simulink model "SingleJoint_Algorithm2"  (R2018b)
settings: Solver=FixedStepDiscrete  StartTime=0.0  StopTime=Inf  FixedStep=0.001  RelTol=1e-3  EnableMultiTasking=on
undefined symbols (not defined in the file): DiscIntNeverNeededParam, J3, J7, Motor_Current, Motor_Position, Motor_Velocity, Send_GUIdata
libraries: c280xlib x14, simulink x7, dspsrcs4 x1, idelinklib_common x1
(part 1 of 2)
settings Model: ExtModeTrigDuration=8  Creator=jeason  LastModifiedBy=Jeason
settings SolverCC: AutoInsertRateTranBlk=on
settings OptimizationCC: DefaultUnderspecifiedDataType=single  EnhancedBackFolding=on  PassReuseOutputArgsAs=Individual arguments  MaxStackSize=512  OptimizeBlockOrder=speed  DifferentSizesBufferReuse=on  OptimizationCustomize=off
settings DebuggingCC: MultiTaskDSMMsg=none  ParameterTunabilityLossMsg=error
settings HardwareCC: ProdBitPerChar=16  ProdBitPerInt=16  ProdBitPerPointer=32  ProdBitPerSizeT=32  ProdBitPerPtrDiffT=32  ProdLargestAtomicInteger=Integer  ProdLargestAtomicFloat=None  ProdWordSize=16  ProdLongLongMode=on  ProdHWDeviceType=Texas Instruments->C2000
settings SFSimCC: MATLABDynamicMemAlloc=off
settings RTWCC: SystemTargetFile=ert.tlc  HardwareBoard=TI Delfino F2833x  TemplateMakefile=ert_default_tmf  GenerateReport=on  Toolchain=Texas Instruments Code Composer Studio (C2000)  IncludeHyperlinkInReport=on  LaunchReport=on  GenerateTraceInfo=on  GenerateTraceReport=on  GenerateTraceReportSl=on  GenerateTraceReportSf=on  GenerateTraceReportEml=on
settings CodeAppCC: ForceParamTrailComments=on  IgnoreCustomStorageClasses=off  OperatorAnnotations=on  SimulinkDataObjDesc=on  SFDataObjDesc=on  InsertBlockDesc=on
settings ERTTargetCC: CodeReplacementLibrary=TI C28x

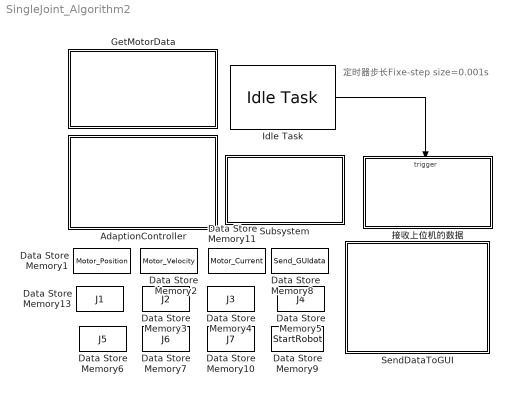
== system SingleJoint_Algorithm2 ==
  note: 定时器步长Fixe-step size=0.001s
  AdaptionController : Subsystem  Tag=Calculated_Data  Priority=1  TreatAsAtomicUnit=on  RTWFcnName=DynamicsController
      settings: RTWSystemCode=Nonreusable function  RTWFcnNameOpts=User specified  RTWFileNameOpts=Use function name
      mask Display:
      | color('red')
      | disp('六轴单关节\n自适应算法2动力学计算')
  Data Store Memory1 : DataStoreMemory  DataStoreName=Motor_Position  ReadBeforeWriteMsg=warning  WriteAfterWriteMsg=warning  WriteAfterReadMsg=warning  InitialValue=[0 0 0 0 0 0]  ShowAdditionalParam=off  OutDataTypeStr=int32
      settings: RTWStateStorageClass=ExportedGlobal
  Data Store Memory10 : DataStoreMemory  DataStoreName=J7  ReadBeforeWriteMsg=warning  WriteAfterWriteMsg=warning  WriteAfterReadMsg=warning  InitialValue=[0 0 0 0 0 0]  ShowAdditionalParam=off  OutDataTypeStr=double
      settings: RTWStateStorageClass=ExportedGlobal
  Data Store Memory11 : DataStoreMemory  DataStoreName=Motor_Current  ReadBeforeWriteMsg=warning  WriteAfterWriteMsg=warning  WriteAfterReadMsg=warning  InitialValue=[0 0 0 0 0 0]  ShowAdditionalParam=off  OutDataTypeStr=int32
      settings: RTWStateStorageClass=ExportedGlobal
  Data Store Memory13 : DataStoreMemory  DataStoreName=J1  ReadBeforeWriteMsg=warning  WriteAfterWriteMsg=warning  WriteAfterReadMsg=warning  InitialValue=[0 0 0 0 0 0]  ShowAdditionalParam=off  OutDataTypeStr=double
      settings: RTWStateStorageClass=ExportedGlobal
  Data Store Memory2 : DataStoreMemory  DataStoreName=Motor_Velocity  ReadBeforeWriteMsg=warning  WriteAfterWriteMsg=warning  WriteAfterReadMsg=warning  InitialValue=[0 0 0 0 0 0]  ShowAdditionalParam=off  OutDataTypeStr=int32
      settings: RTWStateStorageClass=ExportedGlobal
  Data Store Memory3 : DataStoreMemory  DataStoreName=J2  ReadBeforeWriteMsg=warning  WriteAfterWriteMsg=warning  WriteAfterReadMsg=warning  InitialValue=[0 0 0 0 0 0]  ShowAdditionalParam=off  OutDataTypeStr=double
      settings: RTWStateStorageClass=ExportedGlobal
  Data Store Memory4 : DataStoreMemory  DataStoreName=J3  ReadBeforeWriteMsg=warning  WriteAfterWriteMsg=warning  WriteAfterReadMsg=warning  InitialValue=[0 0 0 0 0 0]  ShowAdditionalParam=off  OutDataTypeStr=double
      settings: RTWStateStorageClass=ExportedGlobal
  Data Store Memory5 : DataStoreMemory  DataStoreName=J4  ReadBeforeWriteMsg=warning  WriteAfterWriteMsg=warning  WriteAfterReadMsg=warning  InitialValue=[0 0 0 0 0 0]  ShowAdditionalParam=off  OutDataTypeStr=double
      settings: RTWStateStorageClass=ExportedGlobal
  Data Store Memory6 : DataStoreMemory  DataStoreName=J5  ReadBeforeWriteMsg=warning  WriteAfterWriteMsg=warning  WriteAfterReadMsg=warning  InitialValue=[0 0 0 0 0 0]  ShowAdditionalParam=off  OutDataTypeStr=double
      settings: RTWStateStorageClass=ExportedGlobal
  Data Store Memory7 : DataStoreMemory  DataStoreName=J6  ReadBeforeWriteMsg=warning  WriteAfterWriteMsg=warning  WriteAfterReadMsg=warning  InitialValue=[0 0 0 0 0 0]  ShowAdditionalParam=off  OutDataTypeStr=double
      settings: RTWStateStorageClass=ExportedGlobal
  Data Store Memory8 : DataStoreMemory  DataStoreName=Send_GUIdata  ReadBeforeWriteMsg=warning  WriteAfterWriteMsg=warning  WriteAfterReadMsg=warning  InitialValue=zeros(1,18)  ShowAdditionalParam=off  OutDataTypeStr=double
      settings: RTWStateStorageClass=ExportedGlobal
  Data Store Memory9 : DataStoreMemory  DataStoreName=StartRobot  ReadBeforeWriteMsg=warning  WriteAfterWriteMsg=warning  WriteAfterReadMsg=warning  ShowAdditionalParam=off  OutDataTypeStr=uint16
      settings: RTWStateStorageClass=ExportedGlobal
  GetMotorData : Subsystem  Tag=Get_Data  Priority=0  TreatAsAtomicUnit=on
      settings: RTWSystemCode=Nonreusable function
  Idle Task : idelinklib_common/Idle Task  tasknumbers=[0]  taskpriorities=100016  taskpreempts=[1]  showinput=off  simPriority=0
  SendDataToGUI : Subsystem  Priority=2  TreatAsAtomicUnit=on
      settings: RTWSystemCode=Nonreusable function
  Subsystem : Subsystem
      mask Display: disp('System\nInitialization');
  接收上位机的数据 : Subsystem  TreatAsAtomicUnit=on
  wires:
  Idle Task/1 -> 接收上位机的数据/Trigger

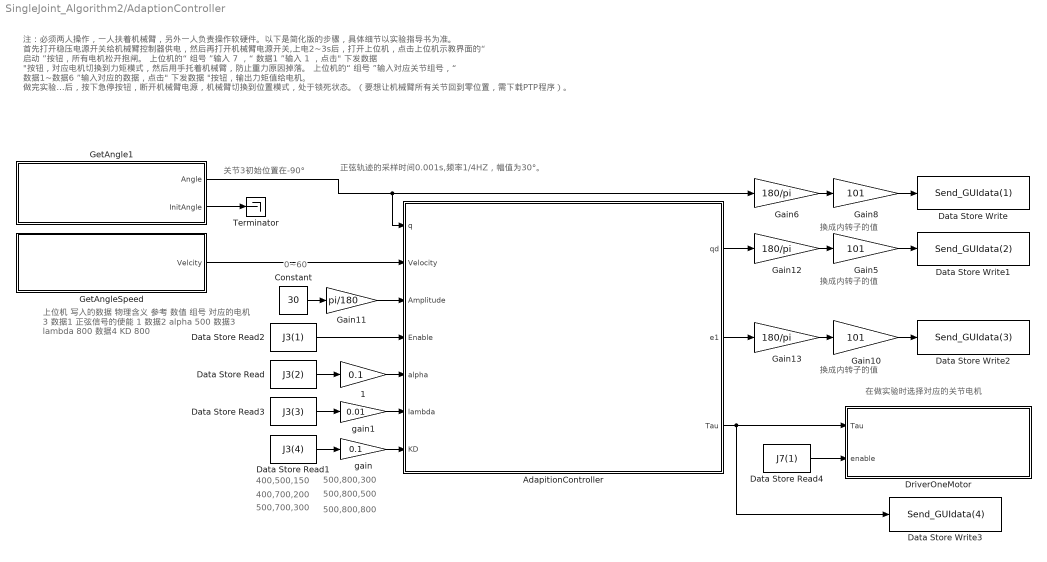
== system SingleJoint_Algorithm2/AdaptionController ==
  note: 400,500,150
  note: 换成内转子的值
  note: 换成内转子的值
  note: 换成内转子的值
  note: 在做实验时选择对应的关节电机
  note: 上位机
      | 写入的数据
      | 物理含义
      | 参考
      | 数值
      |
      | 组号
      | 对应的电机
      | 3
      |
      | 数据1
      | 正弦信号的使能
      | 1
      |
      | 数据2
      | alpha
      | 500
      |
      | 数据3
      | lambda
      | 800
      |
      | 数据4
      | KD
      | 800
  note: 关节3初始位置在-90°
  note: 400,700,200
  note: 500,700,300
  note: 500,800,300
  note: 500,800,800
  note: 注：必须两人操作，一人扶着机械臂，另外一人负责操作软硬件。以下是简化版的步骤，具体细节以实验指导书为准。
      | 首先打开稳压电源开关给机械臂控制器供电，然后再打开机械臂电源开关,上电2~3s后，打开上位机，点击上位机示教界面的“ 启动 ”按钮，所有电机松开抱闸。
      | 上位机的“ 组号 ”输入 7 ，“ 数据1 ”输入 1 ，点击" 下发数据 "按钮，对应电机切换到力矩模式，然后用手托着机械臂，防止重力原因掉落。
      | 上位机的“ 组号 ”输入对应关节组号，“ 数据1~数据6 ”输入对应的数据，点击" 下发数据 "按钮，输出力矩值给电机。
      | 做完实验后，按下急停按钮，断开机械臂电源，机械臂切换到位置模式，处于锁死状态。（要想让机械臂所有关节回到零位置，需下载PTP程序）。
  note: 500,800,500
  note: 正弦轨迹的采样时间0.001s,频率1/4HZ，幅值为30°。
  note: 0~60
  1 : Gain  Gain=0.1  OutDataTypeStr=double
  AdapitionController : Subsystem  Priority=2  TreatAsAtomicUnit=on  RTWFcnName=AdaptiveAlgorithm  mask(单关节自适应算法2控制器){Freq=1/4, SimpleTime=0.001}
      mask prompts: Freq "正弦信号的频率(HZ)"; SimpleTime "正弦信号的采样时间(s)"
      mask help:
      | 采样频率不能过快，否则机械臂摆动频率也会变快，至少为1/4.
      | 采样时间只能是定时器步长的整数倍，否则会报错，正弦信号的幅值最大为pi/3。
      settings: RTWSystemCode=Nonreusable function  RTWFcnNameOpts=User specified  RTWFileNameOpts=Use subsystem name  FunctionInterfaceSpec=Allow arguments
      mask Display:
      | port_label('input', 1, '外转子实际角度(rad)');
      | port_label('input', 2, '外转子实际角速度(rad/s)');
      | port_label('input', 3, '外转子正弦信号的幅值(rad)');
      | port_label('input', 4, '使能信号');
      | port_label('input', 5, 'alpha');
      | port_label('input', 6, 'lambda');
      | port_label('input', 7, 'KD');
      | 
      | port_label('output', 1, '外转子理想正弦信号(rad)');
      | port_label('output', 2, '外转子跟踪误差(rad)');
      | port_label('output', 3, '力矩Tau(N·m)');
  Constant : Constant  Value=30
  Data Store Read : DataStoreRead  DataStoreName=J3  DataStoreElements=J3(2)
  Data Store Read1 : DataStoreRead  DataStoreName=J3  DataStoreElements=J3(4)
  Data Store Read2 : DataStoreRead  DataStoreName=J3  DataStoreElements=J3(1)
  Data Store Read3 : DataStoreRead  DataStoreName=J3  DataStoreElements=J3(3)
  Data Store Read4 : DataStoreRead  DataStoreName=J7  DataStoreElements=J7(1)
  Data Store Write : DataStoreWrite  DataStoreName=Send_GUIdata  DataStoreElements=Send_GUIdata(1)
  Data Store Write1 : DataStoreWrite  DataStoreName=Send_GUIdata  DataStoreElements=Send_GUIdata(2)
  Data Store Write2 : DataStoreWrite  DataStoreName=Send_GUIdata  DataStoreElements=Send_GUIdata(3)
  Data Store Write3 : DataStoreWrite  DataStoreName=Send_GUIdata  DataStoreElements=Send_GUIdata(4)
  DriverOneMotor : Subsystem  TreatAsAtomicUnit=on  mask(驱动单个关节){SelectJoint=3}
      mask prompts: SelectJoint "选择关节电机"
      mask help:
      | 关节1~3为CANB,关节4~6为CANA,驱动的电机的邮箱号统一为7。
      | 输入量的范围限定在-900~900。
      settings: RTWSystemCode=Nonreusable function
      mask TypeOptions SelectJoint: 1 | 2 | 3 | 4 | 5 | 6
      mask Callback SelectJoint:
      | vssBlk1_1 = [gcb, '/BottomDriver/Joint1'];
      | vssBlk1_2 = [gcb, '/BottomDriver/Joint2'];
      | vssBlk1_3 = [gcb, '/BottomDriver/Joint3'];
      | vssBlk1_4 = [gcb, '/BottomDriver/Joint4'];
      | vssBlk1_5 = [gcb, '/BottomDriver/Joint5'];
      | vssBlk1_6 = [gcb, '/BottomDriver/Joint6'];
      | choice1 = get_param(gcb,'SelectJoint');
      | if strcmp(choice1,'1')
      |     set_param(vssBlk1_1, 'Commented','off');
      |     set_param(vssBlk1_2,'Commented','on');
      |     set_param(vssBlk1_3,'Commented','on');
      |     set_param(vssBlk1_4,'Commented','on');
      |     set_param(vssBlk1_5,'Commented','on');
      |     set_param(vssBlk1_6,'Commented','on');
      | elseif strcmp(choice1,'2')
      |     set_param(vssBlk1_2, 'Commented','off');
      |     set_param(vssBlk1_1,'Commented','on');
      |     set_param(vssBlk1_3,'Commented','on');
      |     set_param(vssBlk1_4,'Commented','on');
      |     set_param(vssBlk1_5,'Commented','on');
      |     set_param(vssBlk1_6,'Commented','on');
      | elseif strcmp(choice1,'3')
      |     set_param(vssBlk1_3, 'Commented','off');
      |     set_param(vssBlk1_1,'Commented','on');
      |     set_param(vssBlk1_2,'Commented','on');
      |     set_param(vssBlk1_4,'Commented','on');
      |     set_param(vssBlk1_5,'Commented','on');
      |     set_param(vssBlk1_6,'Commented','on');
      | elseif strcmp(choice1,'4')
      |     set_param(vssBlk1_4, 'Commented','off');
      |     set_param(vssBlk1_1,'Commented','on');
      |     set_param(vssBlk1_2,'Commented','on');
      |     set_param(vssBlk1_3,'Commented','on');
      |     set_param(vssBlk1_5,'Commented','on');
      |     set_param(vssBlk1_6,'Commented','on');
      | elseif strcmp(choice1,'5')
      |     set_param(vssBlk1_5, 'Commented','off');
      |     set_param(vssBlk1_1,'Commented','on');
      |     set_param(vssBlk1_2,'Commented','on');
      |     set_param(vssBlk1_3,'Commented','on');
      |     set_param(vssBlk1_4,'Commented','on');
      |     set_param(vssBlk1_6,'Commented','on');
      | elseif strcmp(choice1,'6')
      |     set_param(vssBlk1_6, 'Commented','off');
      |     set_param(vssBlk1_1,'Commented','on');
      |     set_param(vssBlk1_2,'Commented','on');
      |     set_param(vssBlk1_3,'Commented','on');
      |     set_param(vssBlk1_4,'Commented','on');
      |     set_param(vssBlk1_5,'Commented','on');
      | end
      | clear choice1 vssBlk1_1 vssBlk1_2 vssBlk1_3 vssBlk1_4 vssBlk1_5 vssBlk1_6;
      mask Display:
      | port_label('input', 1, 'Tau');
      | port_label('input', 2, 'Enable');
      | choice1 = get_param(gcb,'SelectJoint');
      | color('black');
      | switch choice1
      |     case '1'
      |         disp('单关节算法\n驱动关节1电机');
      |     case '2'
      |         disp('单关节算法\n驱动关节2电机');
      |     case '3'
      |         disp('单关节算法\n驱动关节3电机');
      |     case '4'
      |         disp('单关节算法\n驱动关节4电机');
      |     case '5'
      |         disp('单关节算法\n驱动关节5电机');
      |     case '6'
      |         disp('单关节算法\n驱动关节6电机');
      | end
      | clear choice1;
  Gain10 : Gain  Gain=101
  Gain11 : Gain  Gain=pi/180
  Gain12 : Gain  Gain=180/pi  OutDataTypeStr=double
  Gain13 : Gain  Gain=180/pi  OutDataTypeStr=double
  Gain5 : Gain  Gain=101
  Gain6 : Gain  Gain=180/pi  OutDataTypeStr=double
  Gain8 : Gain  Gain=101
  GetAngle1 : Subsystem  TreatAsAtomicUnit=on  mask(获取电机外转子角度(rad)){JJoint=3, InitAngle=-90}
      mask prompts: JJoint "选择关节电机"; InitAngle "给定初始角度(deg)"
      mask help:
      | 给定初始角度：假设在数学建模时，设定连杆在水平位置为0°，而机械臂每个关节在出厂时都设定在竖直位置为0°，那么这里就需要给定一个偏置值90°/-90°，默认设为0。
      | 注：关节3因为结构原因实际获取到的角度的正负和标签贴的方向相反。
      | Angle(rad)=电机外转子的实际角度值-给定的初始角度值
      | InitAngle(rad)=给定的初始角度值
      mask TypeOptions JJoint: 1 | 2 | 3 | 4 | 5 | 6
      mask Display:
      | choice1 = get_param(gcb,'JJoint');
      | color('black');
      | switch choice1
      |     case '1'
      |         disp('获取关节1电机\n外转子角度(rad)');
      |     case '2'
      |         disp('获取关节2电机\n外转子角度(rad)');
      |     case '3'
      |         disp('获取关节3电机\n外转子角度(rad)');
      |     case '4'
      |         disp('获取关节4电机\n外转子角度(rad)');
      |     case '5'
      |         disp('获取关节5电机\n外转子角度(rad)');
      |     case '6'
      |         disp('获取关节6电机\n外转子角度(rad)');
      | end
      | color('black');
      | port_label('output', 1, 'Angle');
      | port_label('output', 2, 'InitAngle');
      | clear choice1;
  GetAngleSpeed : Subsystem  Priority=2  TreatAsAtomicUnit=on  mask{JJoint=3}
      mask prompts: JJoint "选择关节电机"
      mask help: 读取电机角速度(rad/s)
      mask TypeOptions JJoint: 1 | 2 | 3 | 4 | 5 | 6
      mask Display:
      | choice1 = get_param(gcb,'JJoint');
      | color('black');
      | switch choice1
      |     case '1'
      |         disp('获取关节1电机\n外转子角速度(rad/s)');
      |     case '2'
      |         disp('获取关节2电机\n外转子角速度(rad/s)');
      |     case '3'
      |         disp('获取关节3电机\n外转子角速度(rad/s)');
      |     case '4'
      |         disp('获取关节4电机\n外转子角速度(rad/s)');
      |     case '5'
      |         disp('获取关节5电机\n外转子角速度(rad/s)');
      |     case '6'
      |         disp('获取关节6电机\n外转子角速度(rad/s)');
      | end
      | color('black');
      | port_label('output', 1, 'Velocity');
      | clear choice1;
  Terminator : Terminator
  gain : Gain  Gain=0.1  OutDataTypeStr=double
  gain1 : Gain  Gain=0.01  OutDataTypeStr=double
  wires:
  GetAngle1/1(Angle) -> AdapitionController/1(q), Gain6/1
  Gain10/1 -> Data Store Write2/1
  Gain5/1 -> Data Store Write1/1
  Data Store Read/1 -> 1/1
  Data Store Read3/1 -> gain1/1
  Data Store Read1/1 -> gain/1
  Gain6/1 -> Gain8/1
  Gain8/1 -> Data Store Write/1
  Constant/1 -> Gain11/1
  Gain12/1 -> Gain5/1
  Gain13/1 -> Gain10/1
  GetAngleSpeed/1(Velcity) -> AdapitionController/2(Velocity)
  1/1 -> AdapitionController/5(alpha)
  Data Store Read2/1 -> AdapitionController/4(Enable)
  Gain11/1 -> AdapitionController/3(Amplitude)
  gain1/1 -> AdapitionController/6(lambda)
  gain/1 -> AdapitionController/7(KD)
  AdapitionController/1(qd) -> Gain12/1
  AdapitionController/2(e1) -> Gain13/1
  Data Store Read4/1 -> DriverOneMotor/2(enable)
  AdapitionController/3(Tau) -> DriverOneMotor/1(Tau), Data Store Write3/1
  GetAngle1/2(InitAngle) -> Terminator/1

== system SingleJoint_Algorithm2/GetMotorData ==
  note: 获取关节电流、 角速度、 角度信息
  CANA_284_24 : Subsystem  Priority=4  TreatAsAtomicUnit=on
      settings: RTWSystemCode=Nonreusable function
      mask Display:
      | color('WHITE')
      | disp('JOINT4\n数据读取')
  CANA_285_25 : Subsystem  Priority=5  TreatAsAtomicUnit=on
      settings: RTWSystemCode=Nonreusable function
      mask Display:
      | color('WHITE')
      | disp('JOINT5\n数据读取')
  CANA_286_26 : Subsystem  Priority=6  TreatAsAtomicUnit=on
      settings: RTWSystemCode=Nonreusable function
      mask Display:
      | color('WHITE')
      | disp('JOINT6\n数据读取')
  CANB_281_21 : Subsystem  Priority=1  TreatAsAtomicUnit=on
      settings: RTWSystemCode=Nonreusable function
      mask Display:
      | color('WHITE')
      | disp('JOINT1\n数据读取')
  CANB_282_22 : Subsystem  Priority=2  TreatAsAtomicUnit=on
      settings: RTWSystemCode=Nonreusable function
      mask Display:
      | color('white')
      | disp('JOINT2\n数据读取')
  CANB_283_23 : Subsystem  Priority=3  TreatAsAtomicUnit=on
      settings: RTWSystemCode=Nonreusable function
      mask Display:
      | color('white')
      | disp('JOINT3\n数据读取')

== system SingleJoint_Algorithm2/SendDataToGUI ==
  note: Upper limit=9
  note: 发送数据给上位机
  note: 定时器步长Fixe-step size=0.001s,
      | 每10ms发送一次数据给上位机
  " " : Subsystem
  Constant : Constant  Value=true  OutDataTypeStr=boolean
  Constant1 : Constant  Value=false  OutDataTypeStr=boolean
  Switch : Switch  Criteria=u2 > Threshold
  广播周期 : simulink/Sources/Counter Limited  uplimit=9  tsamp=-1
  wires:
  Switch/1 -> " "/Enable
  广播周期/1 -> Switch/2
  Constant1/1 -> Switch/1
  Constant/1 -> Switch/3

== system SingleJoint_Algorithm2/Subsystem ==
  Model Header : Subsystem  mask(Model Header){ShowInLibBrowser=0}
      mask prompts: ShowInLibBrowser "Simulink:masks:CustCodeMaskParam1_MP"
      settings: CopyFcn=cccopyfcn(gcb)  OpenFcn=ccopenfcn('Model Header')
      mask Help: eval('feval(''rtwprivate'',''rtwhelpview'',''rtw_model_header_block'')');
      mask Display: disp('Model\nHeader');
  Model Source : Subsystem  mask(Model Source){ShowInLibBrowser=0}
      mask prompts: ShowInLibBrowser "Simulink:masks:CustCodeMaskParam1_MP"
      settings: CopyFcn=cccopyfcn(gcb)  OpenFcn=ccopenfcn('Model Source')
      mask Help: eval('feval(''rtwprivate'',''rtwhelpview'',''rtw_model_source_block'')');
      mask Display: disp('Model\nSource');
  System Initialize : Subsystem  mask(System Initialize){ShowInLibBrowser=0}
      mask prompts: ShowInLibBrowser "Simulink:masks:CustCodeMaskParam1_MP"
      settings: CopyFcn=cccopyfcn(gcb)  OpenFcn=ccopenfcn('System Initialize Function')
      mask Help: eval('feval(''rtwprivate'',''rtwhelpview'',''rtw_sys_initialize_block'')');
      mask Display: disp('System\nInitialize');

== system SingleJoint_Algorithm2/接收上位机的数据 ==
  note: 接收上位机数据
  function : TriggerPort  TriggerType=function-call  VariantControl=Variant
  0x0080 : simulink/Logic and Bit Operations/Compare To Constant  relop===  const=hex2dec('0080')  OutDataTypeStr=boolean
  0x88 : simulink/Logic and Bit Operations/Compare To Constant  relop===  const=hex2dec('0088')  OutDataTypeStr=boolean
  Compare To Constant1 : simulink/Logic and Bit Operations/Compare To Constant  relop===  const=hex2dec('0001')  OutDataTypeStr=boolean
  Compare To Constant2 : simulink/Logic and Bit Operations/Compare To Constant  relop===  const=hex2dec('0001')  OutDataTypeStr=boolean
  Data Store Read : DataStoreRead  DataStoreName=PTX
  Data Store Write2 : DataStoreWrite  DataStoreName=StartRobot
  Data Type Conversion : DataTypeConversion  OutDataTypeStr=int16
  Data Type Conversion3 : DataTypeConversion  OutDataTypeStr=double
  Data Type Conversion4 : DataTypeConversion  OutDataTypeStr=uint16
  Demux1 : Demux  Outputs=9
  Logical Operator : Logic  Inputs=4  AllPortsSameDT=off  OutDataTypeStr=boolean
  Mux1 : Mux  Inputs=6
  Subsystem : Subsystem
  Terminator3 : Terminator
  消息使能 : DataStoreMemory  DataStoreName=PTX  ReadBeforeWriteMsg=warning  WriteAfterWriteMsg=warning  WriteAfterReadMsg=warning  InitialValue=true  ShowAdditionalParam=off  OutDataTypeStr=boolean
  获取用户命令 : Subsystem  Priority=1  TreatAsAtomicUnit=on
      settings: RTWSystemCode=Nonreusable function
  wires:
  Compare To Constant2/1 -> Logical Operator/4
  Compare To Constant1/1 -> Logical Operator/3
  Data Store Read/1 -> Logical Operator/2
  Logical Operator/1 -> Data Type Conversion4/1
  0x0080/1 -> Logical Operator/1
  Demux1/4 -> Mux1/2, Compare To Constant2/1
  Demux1/3 -> Mux1/1, Compare To Constant1/1
  Demux1/1 -> 0x0080/1, 0x88/1
  获取用户命令/1(消息) -> Demux1/1
  Demux1/5 -> Mux1/3
  Demux1/6 -> Mux1/4
  Demux1/9 -> Terminator3/1
  Demux1/7 -> Mux1/5
  Demux1/8 -> Mux1/6
  Mux1/1 -> Data Type Conversion/1
  Data Type Conversion/1 -> Data Type Conversion3/1
  Data Type Conversion4/1 -> Data Store Write2/1
  Demux1/2 -> Subsystem/1(组号)
  Data Type Conversion3/1 -> Subsystem/2(数据)
  0x88/1 -> Subsystem/Enable

== system SingleJoint_Algorithm2/AdaptionController/AdapitionController ==
  q : Inport
  Velocity : Inport  Port=2
  Amplitude : Inport  Port=3
  Enable : Inport  Port=4
  alpha : Inport  Port=5
  lambda : Inport  Port=6
  KD : Inport  Port=7
  Controller : Subsystem  TreatAsAtomicUnit=on
      settings: RTWSystemCode=Nonreusable function
  Error : Subsystem  TreatAsAtomicUnit=on
      settings: RTWSystemCode=Nonreusable function
  Terminator1 : Terminator
  Terminator2 : Terminator
  限幅 : Saturate  UpperLimit=pi/3  LowerLimit=0
  qd : Outport
  e1 : Outport  Port=2
  Tau : Outport  Port=3
  wires:
  Velocity/1 -> Controller/2(velocity), Error/2(velocity)
  Error/2(e1) -> e1/1
  alpha/1 -> Error/5(alpha)
  Error/1(qd) -> qd/1
  Amplitude/1 -> 限幅/1
  Error/6(d_theta_r) -> Terminator1/1
  Error/5(V) -> Terminator2/1
  Enable/1 -> Error/3(enable)
  q/1 -> Controller/1(position), Error/1(q)
  Error/3(dd_theta_r) -> Controller/3(dd_theta_r)
  Error/4(s) -> Controller/4(s)
  lambda/1 -> Controller/5(lambda)
  KD/1 -> Controller/6(KD)
  Controller/1(tau) -> Tau/1
  限幅/1 -> Error/4(gain)

== system SingleJoint_Algorithm2/AdaptionController/DriverOneMotor ==
  note: CAN mbx=7
  Tau : Inport
  enable : Inport  Port=2
  BottomDriver : Subsystem
  Constant1 : Constant  Value=SelectJoint
  Data Store Memory2 : DataStoreMemory  DataStoreName=One_TXD  ReadBeforeWriteMsg=warning  WriteAfterWriteMsg=warning  WriteAfterReadMsg=warning  InitialValue=[0]  ShowAdditionalParam=off  OutDataTypeStr=uint8
      settings: RTWStateStorageClass=ExportedGlobal
  Data Store Read4 : DataStoreRead  DataStoreName=One_TXD
  限幅 : Saturate  UpperLimit=500  LowerLimit=-500
  驱动器指令 : Subsystem  TreatAsAtomicUnit=on
      settings: RTWSystemCode=Nonreusable function
  wires:
  Data Store Read4/1 -> BottomDriver/Enable
  Constant1/1 -> BottomDriver/1(SelectJoint)
  驱动器指令/1(MSG) -> BottomDriver/2(MSG)
  限幅/1 -> 驱动器指令/1(Current)
  Tau/1 -> 限幅/1
  enable/1 -> 驱动器指令/2(enable)

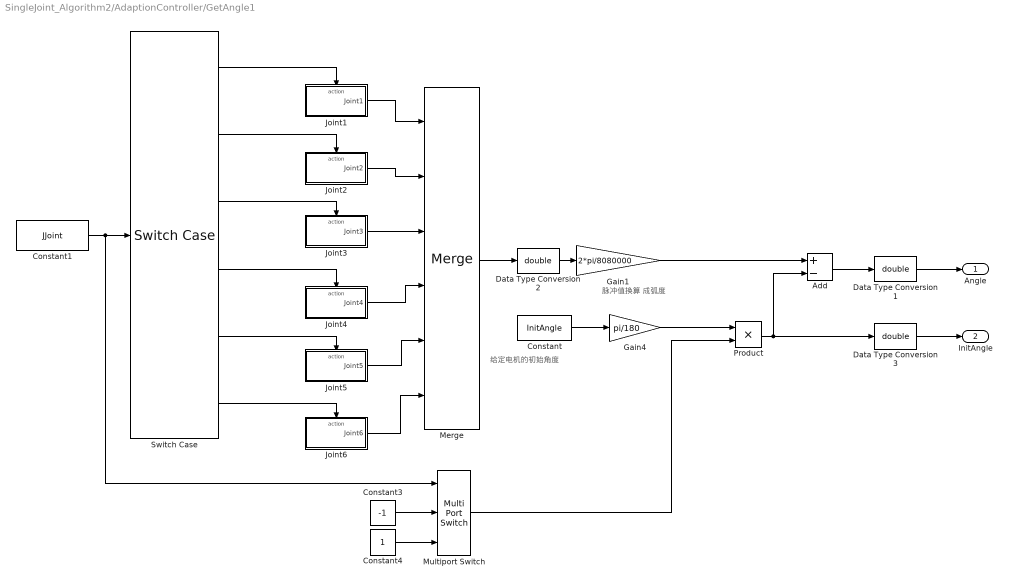
== system SingleJoint_Algorithm2/AdaptionController/GetAngle1 ==
  note: 脉冲值换算
      | 成弧度
  note: 给定电机的初始角度
  Add : Sum  Inputs=+-
  Constant : Constant  Value=InitAngle
  Constant1 : Constant  Value=JJoint  OutDataTypeStr=uint8
  Constant3 : Constant  Value=-1
  Constant4 : Constant
  Data Type Conversion1 : DataTypeConversion  OutDataTypeStr=double
  Data Type Conversion2 : DataTypeConversion  OutDataTypeStr=double
  Data Type Conversion3 : DataTypeConversion  OutDataTypeStr=double
  Gain1 : Gain  Gain=2*pi/8080000
  Gain4 : Gain  Gain=pi/180
  Joint1 : Subsystem  TreatAsAtomicUnit=on
  Joint2 : Subsystem  TreatAsAtomicUnit=on
  Joint3 : Subsystem  TreatAsAtomicUnit=on
  Joint4 : Subsystem  TreatAsAtomicUnit=on
  Joint5 : Subsystem  TreatAsAtomicUnit=on
  Joint6 : Subsystem  TreatAsAtomicUnit=on
  Merge : Merge  Inputs=6  InitialOutput=0
  Multiport Switch : MultiPortSwitch  DataPortOrder=Specify indices  Inputs=2  DataPortIndices={3,[1,2,4,5,6]}
  Product : Product
  Switch Case : SwitchCase  CaseConditions={1 2 3 4 5 6}  ShowDefaultCase=off
  Angle : Outport
  InitAngle : Outport  Port=2
  wires:
  Data Type Conversion2/1 -> Gain1/1
  Data Type Conversion1/1 -> Angle/1
  Joint6/1(Joint6) -> Merge/6
  Joint5/1(Joint5) -> Merge/5
  Joint4/1(Joint4) -> Merge/4
  Joint3/1(Joint3) -> Merge/3
  Joint2/1(Joint2) -> Merge/2
  Joint1/1(Joint1) -> Merge/1
  Switch Case/6 -> Joint6/Action
  Switch Case/5 -> Joint5/Action
  Switch Case/4 -> Joint4/Action
  Switch Case/3 -> Joint3/Action
  Switch Case/2 -> Joint2/Action
  Switch Case/1 -> Joint1/Action
  Constant/1 -> Gain4/1
  Add/1 -> Data Type Conversion1/1
  Gain1/1 -> Add/1
  Gain4/1 -> Product/1
  Merge/1 -> Data Type Conversion2/1
  Multiport Switch/1 -> Product/2
  Constant4/1 -> Multiport Switch/3
  Constant3/1 -> Multiport Switch/2
  Constant1/1 -> Multiport Switch/1, Switch Case/1
  Product/1 -> Data Type Conversion3/1, Add/2
  Data Type Conversion3/1 -> InitAngle/1

== system SingleJoint_Algorithm2/AdaptionController/GetAngleSpeed ==
  note: 换算成角速度2π/1min
  Constant1 : Constant  Value=JJoint
  Data Type Conversion3 : DataTypeConversion  OutDataTypeStr=double
  Gain3 : Gain  Gain=2*pi/60
  Gain9 : Gain  Gain=1/101
  Joint1 : Subsystem  TreatAsAtomicUnit=on
  Joint2 : Subsystem  TreatAsAtomicUnit=on
  Joint3 : Subsystem  TreatAsAtomicUnit=on
  Joint4 : Subsystem  TreatAsAtomicUnit=on
  Joint5 : Subsystem  TreatAsAtomicUnit=on
  Joint6 : Subsystem  TreatAsAtomicUnit=on
  Merge1 : Merge  Inputs=6  InitialOutput=0
  Switch Case : SwitchCase  CaseConditions={1 2 3 4 5 6}  ShowDefaultCase=off
  Velcity : Outport
  wires:
  Constant1/1 -> Switch Case/1
  Switch Case/1 -> Joint1/Action
  Switch Case/2 -> Joint2/Action
  Switch Case/3 -> Joint3/Action
  Switch Case/4 -> Joint4/Action
  Switch Case/5 -> Joint5/Action
  Switch Case/6 -> Joint6/Action
  Data Type Conversion3/1 -> Gain3/1
  Joint6/1(Joint6_Velocity) -> Merge1/6
  Joint5/1(Joint5_Velocity) -> Merge1/5
  Joint4/1(Joint4_Velocity) -> Merge1/4
  Joint3/1(Joint3_Velocity) -> Merge1/3
  Joint2/1(Joint2_Velocity) -> Merge1/2
  Joint1/1(Joint1_Velocity) -> Merge1/1
  Gain3/1 -> Gain9/1
  Gain9/1 -> Velcity/1
  Merge1/1 -> Data Type Conversion3/1

== system SingleJoint_Algorithm2/GetMotorData/CANA_284_24 ==
  note: 控制器接收ID:0x280+“ID”
  Subsystem1 : Subsystem
  eCAN Receive1 : c280xlib/eCAN Receive  chipFamily=C280x  useModule=eCAN_A  mailboxNo=24  messageID=hex2dec('284')  messageType=Standard (11-bit identifier)  sampleTime=-1  dataType=uint8  initValue=0  outputMessageLength=off  outputMessageTimeStamp=off  postInterrupt=off  interruptLine=0
      settings: SourceProductName=Embedded Coder Support Package for Texas Instruments C2000 Processors  SourceProductBaseCode=TIC2000
  wires:
  eCAN Receive1/2 -> Subsystem1/1(In1)
  eCAN Receive1/1 -> Subsystem1/Trigger

== system SingleJoint_Algorithm2/GetMotorData/CANA_285_25 ==
  note: 控制器接收ID:0x280+“ID”
  Subsystem : Subsystem
  eCAN Receive : c280xlib/eCAN Receive  chipFamily=C280x  useModule=eCAN_A  mailboxNo=25  messageID=hex2dec('285')  messageType=Standard (11-bit identifier)  sampleTime=-1  dataType=uint8  initValue=0  outputMessageLength=off  outputMessageTimeStamp=off  postInterrupt=off  interruptLine=0
      settings: SourceProductName=Embedded Coder Support Package for Texas Instruments C2000 Processors  SourceProductBaseCode=TIC2000
  wires:
  eCAN Receive/2 -> Subsystem/1(In1)
  eCAN Receive/1 -> Subsystem/Trigger

== system SingleJoint_Algorithm2/GetMotorData/CANA_286_26 ==
  note: 控制器接收ID:0x280+“ID”
  Subsystem : Subsystem
  eCAN Receive : c280xlib/eCAN Receive  chipFamily=C280x  useModule=eCAN_A  mailboxNo=26  messageID=hex2dec('286')  messageType=Standard (11-bit identifier)  sampleTime=-1  dataType=uint8  initValue=0  outputMessageLength=off  outputMessageTimeStamp=off  postInterrupt=off  interruptLine=0
      settings: SourceProductName=Embedded Coder Support Package for Texas Instruments C2000 Processors  SourceProductBaseCode=TIC2000
  wires:
  eCAN Receive/2 -> Subsystem/1(In1)
  eCAN Receive/1 -> Subsystem/Trigger

== system SingleJoint_Algorithm2/GetMotorData/CANB_281_21 ==
  note: 控制器接收ID:0x280+“ID”
  Subsystem : Subsystem
  eCAN Receive : c280xlib/eCAN Receive  chipFamily=C280x  useModule=eCAN_B  mailboxNo=21  messageID=hex2dec('281')  messageType=Standard (11-bit identifier)  sampleTime=-1  dataType=uint8  initValue=0  outputMessageLength=off  outputMessageTimeStamp=off  postInterrupt=off  interruptLine=0
      settings: SourceProductName=Embedded Coder Support Package for Texas Instruments C2000 Processors  SourceProductBaseCode=TIC2000
  wires:
  eCAN Receive/2 -> Subsystem/1(In1)
  eCAN Receive/1 -> Subsystem/Trigger

== system SingleJoint_Algorithm2/GetMotorData/CANB_282_22 ==
  note: 控制器接收ID:0x280+“ID”
  Subsystem : Subsystem
  eCAN Receive : c280xlib/eCAN Receive  chipFamily=C280x  useModule=eCAN_B  mailboxNo=22  messageID=hex2dec('282')  messageType=Standard (11-bit identifier)  sampleTime=-1  dataType=uint8  initValue=0  outputMessageLength=off  outputMessageTimeStamp=off  postInterrupt=off  interruptLine=0
      settings: SourceProductName=Embedded Coder Support Package for Texas Instruments C2000 Processors  SourceProductBaseCode=TIC2000
  wires:
  eCAN Receive/2 -> Subsystem/1(In1)
  eCAN Receive/1 -> Subsystem/Trigger

== system SingleJoint_Algorithm2/GetMotorData/CANB_283_23 ==
  note: 控制器接收ID:0x280+“ID”
  Subsystem : Subsystem
  eCAN Receive : c280xlib/eCAN Receive  chipFamily=C280x  useModule=eCAN_B  mailboxNo=23  messageID=hex2dec('283')  messageType=Standard (11-bit identifier)  sampleTime=-1  dataType=uint8  initValue=0  outputMessageLength=off  outputMessageTimeStamp=off  postInterrupt=off  interruptLine=0
      settings: SourceProductName=Embedded Coder Support Package for Texas Instruments C2000 Processors  SourceProductBaseCode=TIC2000
  wires:
  eCAN Receive/2 -> Subsystem/1(In1)
  eCAN Receive/1 -> Subsystem/Trigger

== system SingleJoint_Algorithm2/SendDataToGUI/  ==
  Enable : EnablePort
  Constant1 : Constant  Value=hex2dec('5a')  OutDataTypeStr=uint16
  Data Store Read4 : DataStoreRead  DataStoreName=Send_GUIdata
  Data Type Conversion12 : DataTypeConversion  OutDataTypeStr=uint16
  Demux : Demux  Outputs=18
  Mux : Mux  Inputs=20
  SCI Transmit : c280xlib/SCI Transmit  sciModule=A  dataHead=''  dataTail=''  postInterrupt=off  numFifo=1
      settings: SourceProductName=Embedded Coder Support Package for Texas Instruments C2000 Processors
  校验码填充 : Sum  Inputs=+++++++++++++++++++  AccumDataTypeStr=uint16
  wires:
  Demux/1 -> Mux/2, 校验码填充/2
  Mux/1 -> SCI Transmit/1
  Demux/3 -> 校验码填充/4, Mux/4
  Demux/14 -> 校验码填充/15, Mux/15
  Demux/9 -> 校验码填充/10, Mux/10
  Demux/5 -> Mux/6, 校验码填充/6
  Demux/2 -> 校验码填充/3, Mux/3
  Data Store Read4/1 -> Data Type Conversion12/1
  Demux/13 -> 校验码填充/14, Mux/14
  Demux/6 -> Mux/7, 校验码填充/7
  Demux/8 -> 校验码填充/9, Mux/9
  Demux/10 -> 校验码填充/11, Mux/11
  Demux/4 -> 校验码填充/5, Mux/5
  Demux/7 -> 校验码填充/8, Mux/8
  Demux/15 -> 校验码填充/16, Mux/16
  Demux/11 -> 校验码填充/12, Mux/12
  Demux/18 -> 校验码填充/19, Mux/19
  Demux/16 -> 校验码填充/17, Mux/17
  Constant1/1 -> 校验码填充/1, Mux/1
  Demux/17 -> 校验码填充/18, Mux/18
  校验码填充/1 -> Mux/20
  Demux/12 -> 校验码填充/13, Mux/13
  Data Type Conversion12/1 -> Demux/1

== system SingleJoint_Algorithm2/Subsystem/Model Header ==

== system SingleJoint_Algorithm2/Subsystem/Model Source ==

== system SingleJoint_Algorithm2/Subsystem/System Initialize ==

== system SingleJoint_Algorithm2/接收上位机的数据/Subsystem ==
  组号 : Inport
  数据 : Inport  Port=2
  Enable : EnablePort
  Joint1 : Subsystem  TreatAsAtomicUnit=on
  Joint2 : Subsystem  TreatAsAtomicUnit=on
  Joint3 : Subsystem  TreatAsAtomicUnit=on
  Joint4 : Subsystem  TreatAsAtomicUnit=on
  Joint5 : Subsystem  TreatAsAtomicUnit=on
  Joint6 : Subsystem  TreatAsAtomicUnit=on
  Joint7 : Subsystem  TreatAsAtomicUnit=on
  Switch Case : SwitchCase  CaseConditions={1 2 3 4 5 6 7}  ShowDefaultCase=off
  wires:
  数据/1 -> Joint7/1(Joint7), Joint5/1(Joint5), Joint4/1(Joint4), Joint3/1(Joint3), Joint2/1(Joint2), Joint1/1(Joint1), Joint6/1(Joint6)
  Switch Case/5 -> Joint5/Action
  Switch Case/6 -> Joint6/Action
  Switch Case/2 -> Joint2/Action
  Switch Case/1 -> Joint1/Action
  Switch Case/3 -> Joint3/Action
  Switch Case/4 -> Joint4/Action
  组号/1 -> Switch Case/1
  Switch Case/7 -> Joint7/Action

== system SingleJoint_Algorithm2/接收上位机的数据/获取用户命令 ==
  " " : c280xlib/SCI Receive  sciModule=A  dataHead=''  dataTail=''  dataType=uint16  dataDim=9  initValue=0  errOption=Output the last received value  errValue=0  sampleTime=-1  outputStatus=on  postInterrupt=off  numFifo=1
      settings: SourceProductName=Embedded Coder Support Package for Texas Instruments C2000 Processors  SourceProductBaseCode=TIC2000
  Constant : Constant  Value=false  OutDataTypeStr=boolean
  Constant1 : Constant  Value=true  OutDataTypeStr=boolean
  Data Store Write1 : DataStoreWrite  DataStoreName=PTX
  Logical Operator : Logic  AllPortsSameDT=off  OutDataTypeStr=boolean
  Switch : Switch  Criteria=u2 > Threshold
  消息校验 : Subsystem
  消息 : Outport
  wires:
  消息校验/2(使能) -> Logical Operator/1
  Switch/1 -> Logical Operator/2
  Constant1/1 -> Switch/3
  " "/2 -> Switch/2
  消息校验/1(消息) -> 消息/1
  " "/1 -> 消息校验/1(数据)
  Logical Operator/1 -> Data Store Write1/1
  Constant/1 -> Switch/1

== system SingleJoint_Algorithm2/AdaptionController/AdapitionController/Controller ==
  note: $\dot \eta_2=F\eta_2+HY(\theta,\dot\theta,\ddot\theta_r)+FHY_J(s)$
  note: $\dot \eta_1=F\eta_1+H\tau$
  note: $\tau=f\hat\omega+\Gamma_0\eta_1-K_Ds$
  note: 延时一个采样周期
  position : Inport
  velocity : Inport  Port=2
  dd_theta_r : Inport  Port=3
  s : Inport  Port=4
  lambda : Inport  Port=5
  KD : Inport  Port=6
  Discrete-Time Integrator1 : DiscreteIntegrator  SampleTime=-1  LimitOutput=on  UpperSaturationLimit=[1000 1000 1000;1000 1000 1000;1000 1000 1000;]  LowerSaturationLimit=[-1000 -1000 -1000;-1000 -1000 -1000;-1000 -1000 -1000;]  ICPrevOutput=DiscIntNeverNeededParam  ICPrevScaledInput=DiscIntNeverNeededParam
  Discrete-Time Integrator3 : DiscreteIntegrator  SampleTime=-1  LimitOutput=on  UpperSaturationLimit=[1000;1000;1000;]  LowerSaturationLimit=[-1000;-1000;-1000;]  ICPrevOutput=DiscIntNeverNeededParam  ICPrevScaledInput=DiscIntNeverNeededParam
  SolveTau : Subsystem  TreatAsAtomicUnit=on
      settings: RTWSystemCode=Nonreusable function  FunctionInterfaceSpec=Allow arguments
  Unit Delay : UnitDelay  SampleTime=-1
  Unit Delay1 : UnitDelay  SampleTime=-1
  Unit Delay2 : UnitDelay  SampleTime=-1
  adaptive : Subsystem  TreatAsAtomicUnit=on
      settings: RTWSystemCode=Nonreusable function  FunctionInterfaceSpec=Allow arguments
  im1 : Subsystem  TreatAsAtomicUnit=on
      settings: RTWSystemCode=Nonreusable function  FunctionInterfaceSpec=Allow arguments
  im2 : Subsystem  TreatAsAtomicUnit=on
      settings: RTWSystemCode=Nonreusable function  FunctionInterfaceSpec=Allow arguments
  tau : Outport
  wires:
  im2/1(d_eta2) -> Discrete-Time Integrator1/1
  Unit Delay1/1 -> adaptive/1(eta1), im1/2(eta1)
  s/1 -> im2/4(s), SolveTau/5(s), adaptive/6(s)
  dd_theta_r/1 -> im2/3(dd_theta_r), adaptive/5(dd_theta_r)
  position/1 -> adaptive/3(theta), im2/1(position)
  Discrete-Time Integrator1/1 -> Unit Delay2/1
  Discrete-Time Integrator3/1 -> Unit Delay1/1
  Unit Delay/1 -> im1/1(tau)
  im1/1(d_eta1) -> Discrete-Time Integrator3/1
  Unit Delay2/1 -> adaptive/2(eta2), im2/5(eta2)
  velocity/1 -> adaptive/4(d_theta), im2/2(d_theta)
  SolveTau/1(Tau) -> Unit Delay/1, tau/1
  adaptive/1(Gamma0 eta1) -> SolveTau/1(Gamma0 eta1)
  adaptive/2(f) -> SolveTau/2(f)
  lambda/1 -> SolveTau/3(lambda)
  KD/1 -> SolveTau/4(KD)

== system SingleJoint_Algorithm2/AdaptionController/AdapitionController/Error ==
  note: 期望速度
  note: 期望位置
  note: $s(t)=\alpha e_1(t)+e_2(t)$
  note: $\dot\theta_r(t)=\dot\theta_d(t)-\alpha e_1(t)$
  note: $\ddot\theta_r(t)=\ddot\theta_d(t)-\alpha e_2(t)$
  note: $e_2(t)=\dot\theta(t)-\dot\theta_d(t)$
  q : Inport
  velocity : Inport  Port=2
  enable : Inport  Port=3
  gain : Inport  Port=4
  alpha : Inport  Port=5
  Discrete Derivative : simulink/Discrete/Discrete Derivative  gainval=1.0  ICPrevScaledInput=0.0  OutMin=[]  OutMax=[]  OutDataType=fixdt(1, 16)  OutScaling=2^-10  DoSatur=off
  Discrete Derivative1 : simulink/Discrete/Discrete Derivative  gainval=1.0  ICPrevScaledInput=0.0  OutMin=[]  OutMax=[]  OutDataType=fixdt(1, 16)  OutScaling=2^-10  DoSatur=off
  Product1 : Product
  Product5 : Product
  Subsystem : Subsystem
  Sum1 : Sum  Inputs=|-+
  Sum2 : Sum  Inputs=|-+
  Sum3 : Sum  Inputs=|-+
  Sum4 : Sum  Inputs=++|
  qd : Outport
  e1 : Outport  Port=2
  dd_theta_r : Outport  Port=3
  s : Outport  Port=4
  V : Outport  Port=5
  d_theta_r : Outport  Port=6
  wires:
  velocity/1 -> Sum1/2
  Product1/1 -> Sum4/1, Sum2/1
  Sum1/1 -> Product5/2, Sum4/2
  Product5/1 -> Sum3/1
  Sum2/1 -> d_theta_r/1
  Sum3/1 -> dd_theta_r/1
  Sum4/1 -> s/1
  enable/1 -> Subsystem/Enable
  Discrete Derivative/1 -> Sum2/2, V/1, Sum1/1, Discrete Derivative1/1
  Discrete Derivative1/1 -> Sum3/2
  alpha/1 -> Product1/2, Product5/1
  Subsystem/2(qd) -> qd/1, Discrete Derivative/1
  Subsystem/1(e1) -> e1/1, Product1/1
  q/1 -> Subsystem/1(q1)
  gain/1 -> Subsystem/2(gian)

== system SingleJoint_Algorithm2/AdaptionController/DriverOneMotor/BottomDriver ==
  SelectJoint : Inport
  MSG : Inport  Port=2
  Enable : EnablePort
  Joint1 : Subsystem  Commented=on  TreatAsAtomicUnit=on
  Joint2 : Subsystem  Commented=on  TreatAsAtomicUnit=on
  Joint3 : Subsystem  TreatAsAtomicUnit=on
  Joint4 : Subsystem  Commented=on  TreatAsAtomicUnit=on
  Joint5 : Subsystem  Commented=on  TreatAsAtomicUnit=on
  Joint6 : Subsystem  Commented=on  TreatAsAtomicUnit=on
  Switch Case : SwitchCase  CaseConditions={1 2 3 4 5 6}  ShowDefaultCase=off
  wires:
  SelectJoint/1 -> Switch Case/1
  Switch Case/6 -> Joint6/Action
  Switch Case/4 -> Joint4/Action
  Switch Case/2 -> Joint2/Action
  Switch Case/1 -> Joint1/Action
  Switch Case/3 -> Joint3/Action
  Switch Case/5 -> Joint5/Action
  MSG/1 -> Joint1/1(In6), Joint3/1(In1), Joint6/1(In1), Joint5/1(In1), Joint4/1(In1), Joint2/1(In1)

== system SingleJoint_Algorithm2/AdaptionController/DriverOneMotor/驱动器指令 ==
  Current : Inport
  enable : Inport  Port=2
  Data Store Read : DataStoreRead  DataStoreName=StartRobot
  Data Type Conversion1 : DataTypeConversion  OutDataTypeStr=uint8
  Data Type Conversion4 : DataTypeConversion  OutDataTypeStr=uint16
  Data Type Conversion7 : DataTypeConversion  OutDataTypeStr=uint16
  DriveOder : Stateflow chart  TreatAsAtomicUnit=on
  MSG : Outport  OutDataTypeStr=uint8
  wires:
  Data Type Conversion7/1 -> DriveOder/1(Current)
  Current/1 -> Data Type Conversion7/1
  DriveOder/1(MSG) -> Data Type Conversion1/1
  Data Type Conversion1/1 -> MSG/1
  Data Store Read/1 -> DriveOder/2(StartRobot)
  Data Type Conversion4/1 -> DriveOder/3(write)
  enable/1 -> Data Type Conversion4/1

== system SingleJoint_Algorithm2/AdaptionController/GetAngle1/Joint1 ==
  note: 内转子位置的脉冲值
  Action Port : ActionPort
  Data Store Read5 : DataStoreRead  DataStoreName=Motor_Position  DataStoreElements=Motor_Position(1)
  Joint1 : Outport
  wires:
  Data Store Read5/1 -> Joint1/1

== system SingleJoint_Algorithm2/AdaptionController/GetAngle1/Joint2 ==
  Action Port : ActionPort
  Data Store Read5 : DataStoreRead  DataStoreName=Motor_Position  DataStoreElements=Motor_Position(2)
  Joint2 : Outport
  wires:
  Data Store Read5/1 -> Joint2/1

== system SingleJoint_Algorithm2/AdaptionController/GetAngle1/Joint3 ==
  Action Port : ActionPort
  Data Store Read5 : DataStoreRead  DataStoreName=Motor_Position  DataStoreElements=Motor_Position(3)
  Joint3 : Outport
  wires:
  Data Store Read5/1 -> Joint3/1

== system SingleJoint_Algorithm2/AdaptionController/GetAngle1/Joint4 ==
  Action Port : ActionPort
  Data Store Read5 : DataStoreRead  DataStoreName=Motor_Position  DataStoreElements=Motor_Position(4)
  Joint4 : Outport
  wires:
  Data Store Read5/1 -> Joint4/1

== system SingleJoint_Algorithm2/AdaptionController/GetAngle1/Joint5 ==
  Action Port : ActionPort
  Data Store Read5 : DataStoreRead  DataStoreName=Motor_Position  DataStoreElements=Motor_Position(5)
  Joint5 : Outport
  wires:
  Data Store Read5/1 -> Joint5/1

== system SingleJoint_Algorithm2/AdaptionController/GetAngle1/Joint6 ==
  Action Port : ActionPort
  Data Store Read5 : DataStoreRead  DataStoreName=Motor_Position  DataStoreElements=Motor_Position(6)
  Joint6 : Outport
  wires:
  Data Store Read5/1 -> Joint6/1

== system SingleJoint_Algorithm2/AdaptionController/GetAngleSpeed/Joint1 ==
  note: 内转子速度
      | 的脉冲值
  Action Port : ActionPort  ActionType=case
  Data Store Read1 : DataStoreRead  DataStoreName=Motor_Velocity  DataStoreElements=Motor_Velocity(1)
  Joint1_Velocity : Outport
  wires:
  Data Store Read1/1 -> Joint1_Velocity/1

== system SingleJoint_Algorithm2/AdaptionController/GetAngleSpeed/Joint2 ==
  note: 内转子速度
      | 的脉冲值
  Action Port : ActionPort  ActionType=case
  Data Store Read1 : DataStoreRead  DataStoreName=Motor_Velocity  DataStoreElements=Motor_Velocity(2)
  Joint2_Velocity : Outport
  wires:
  Data Store Read1/1 -> Joint2_Velocity/1

== system SingleJoint_Algorithm2/AdaptionController/GetAngleSpeed/Joint3 ==
  note: 内转子速度
      | 的脉冲值
  Action Port : ActionPort  ActionType=case
  Data Store Read1 : DataStoreRead  DataStoreName=Motor_Velocity  DataStoreElements=Motor_Velocity(3)
  Joint3_Velocity : Outport
  wires:
  Data Store Read1/1 -> Joint3_Velocity/1

== system SingleJoint_Algorithm2/AdaptionController/GetAngleSpeed/Joint4 ==
  note: 内转子速度
      | 的脉冲值
  Action Port : ActionPort  ActionType=case
  Data Store Read1 : DataStoreRead  DataStoreName=Motor_Velocity  DataStoreElements=Motor_Velocity(4)
  Joint4_Velocity : Outport
  wires:
  Data Store Read1/1 -> Joint4_Velocity/1

== system SingleJoint_Algorithm2/AdaptionController/GetAngleSpeed/Joint5 ==
  note: 内转子速度
      | 的脉冲值
  Action Port : ActionPort  ActionType=case
  Data Store Read1 : DataStoreRead  DataStoreName=Motor_Velocity  DataStoreElements=Motor_Velocity(5)
  Joint5_Velocity : Outport
  wires:
  Data Store Read1/1 -> Joint5_Velocity/1

== system SingleJoint_Algorithm2/AdaptionController/GetAngleSpeed/Joint6 ==
  note: 内转子速度
      | 的脉冲值
  Action Port : ActionPort  ActionType=case
  Data Store Read1 : DataStoreRead  DataStoreName=Motor_Velocity  DataStoreElements=Motor_Velocity(6)
  Joint6_Velocity : Outport
  wires:
  Data Store Read1/1 -> Joint6_Velocity/1

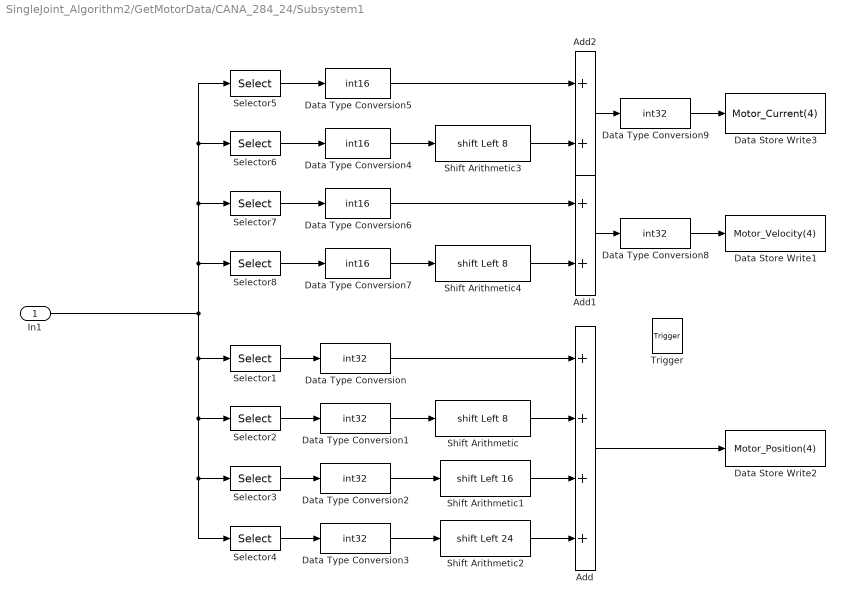
== system SingleJoint_Algorithm2/GetMotorData/CANA_284_24/Subsystem1 ==
  In1 : Inport
  Trigger : TriggerPort  TriggerType=function-call  VariantControl=Variant  PortDimensions=1
  Add : Sum  Inputs=4
  Add1 : Sum  Inputs=2
  Add2 : Sum  Inputs=2
  Data Store Write1 : DataStoreWrite  DataStoreName=Motor_Velocity  DataStoreElements=Motor_Velocity(4)
  Data Store Write2 : DataStoreWrite  DataStoreName=Motor_Position  DataStoreElements=Motor_Position(4)
  Data Store Write3 : DataStoreWrite  DataStoreName=Motor_Current  DataStoreElements=Motor_Current(4)
  Data Type Conversion{,1..3,8..9} (6 alike) : DataTypeConversion  OutDataTypeStr=int32
  Data Type Conversion{4..7} (4 alike) : DataTypeConversion  OutDataTypeStr=int16
  Selector1 : Selector  IndexMode=Zero-based  InputPortWidth=8  IndexOptions=Index vector (dialog)  Indices=4  OutputSizes=1
  Selector2 : Selector  IndexMode=Zero-based  InputPortWidth=8  IndexOptions=Index vector (dialog)  Indices=5  OutputSizes=1
  Selector3 : Selector  IndexMode=Zero-based  InputPortWidth=8  IndexOptions=Index vector (dialog)  Indices=6  OutputSizes=1
  Selector4 : Selector  IndexMode=Zero-based  InputPortWidth=8  IndexOptions=Index vector (dialog)  Indices=7  OutputSizes=1
  Selector5 : Selector  IndexMode=Zero-based  InputPortWidth=8  IndexOptions=Index vector (dialog)  Indices=0  OutputSizes=1
  Selector6 : Selector  IndexMode=Zero-based  InputPortWidth=8  IndexOptions=Index vector (dialog)  Indices=1  OutputSizes=1
  Selector7 : Selector  IndexMode=Zero-based  InputPortWidth=8  IndexOptions=Index vector (dialog)  Indices=2  OutputSizes=1
  Selector8 : Selector  IndexMode=Zero-based  InputPortWidth=8  IndexOptions=Index vector (dialog)  Indices=3  OutputSizes=1
  Shift Arithmetic : ArithShift  BitShiftNumber=8  BitShiftDirection=Left
  Shift Arithmetic1 : ArithShift  BitShiftNumber=16  BitShiftDirection=Left
  Shift Arithmetic2 : ArithShift  BitShiftNumber=24  BitShiftDirection=Left
  Shift Arithmetic3 : ArithShift  BitShiftNumber=8  BitShiftDirection=Left
  Shift Arithmetic4 : ArithShift  BitShiftNumber=8  BitShiftDirection=Left
  wires:
  Selector3/1 -> Data Type Conversion2/1
  Shift Arithmetic/1 -> Add/2
  Shift Arithmetic2/1 -> Add/4
  Data Type Conversion/1 -> Add/1
  Selector1/1 -> Data Type Conversion/1
  Selector4/1 -> Data Type Conversion3/1
  Add/1 -> Data Store Write2/1
  Shift Arithmetic1/1 -> Add/3
  Selector2/1 -> Data Type Conversion1/1
  Data Type Conversion7/1 -> Shift Arithmetic4/1
  Data Type Conversion6/1 -> Add1/1
  Selector7/1 -> Data Type Conversion6/1
  Selector8/1 -> Data Type Conversion7/1
  Selector6/1 -> Data Type Conversion4/1
  In1/1 -> Selector3/1, Selector4/1, Selector2/1, Selector1/1, Selector5/1, Selector6/1, Selector7/1, Selector8/1
  Add1/1 -> Data Type Conversion8/1
  Shift Arithmetic4/1 -> Add1/2
  Data Type Conversion1/1 -> Shift Arithmetic/1
  Data Type Conversion2/1 -> Shift Arithmetic1/1
  Data Type Conversion3/1 -> Shift Arithmetic2/1
  Selector5/1 -> Data Type Conversion5/1
  Data Type Conversion4/1 -> Shift Arithmetic3/1
  Data Type Conversion8/1 -> Data Store Write1/1
  Shift Arithmetic3/1 -> Add2/2
  Data Type Conversion5/1 -> Add2/1
  Add2/1 -> Data Type Conversion9/1
  Data Type Conversion9/1 -> Data Store Write3/1

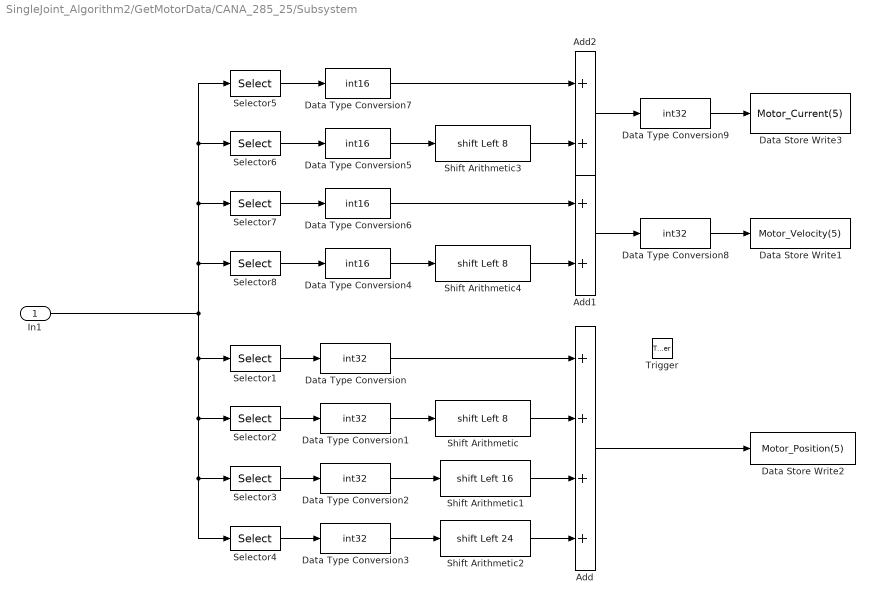
== system SingleJoint_Algorithm2/GetMotorData/CANA_285_25/Subsystem ==
  In1 : Inport
  Trigger : TriggerPort  TriggerType=function-call  VariantControl=Variant  PortDimensions=1
  Add : Sum  Inputs=4
  Add1 : Sum  Inputs=2
  Add2 : Sum  Inputs=2
  Data Store Write1 : DataStoreWrite  DataStoreName=Motor_Velocity  DataStoreElements=Motor_Velocity(5)
  Data Store Write2 : DataStoreWrite  DataStoreName=Motor_Position  DataStoreElements=Motor_Position(5)
  Data Store Write3 : DataStoreWrite  DataStoreName=Motor_Current  DataStoreElements=Motor_Current(5)
  Data Type Conversion{,1..3,8..9} (6 alike) : DataTypeConversion  OutDataTypeStr=int32
  Data Type Conversion{4..7} (4 alike) : DataTypeConversion  OutDataTypeStr=int16
  Selector1 : Selector  IndexMode=Zero-based  InputPortWidth=8  IndexOptions=Index vector (dialog)  Indices=4  OutputSizes=1
  Selector2 : Selector  IndexMode=Zero-based  InputPortWidth=8  IndexOptions=Index vector (dialog)  Indices=5  OutputSizes=1
  Selector3 : Selector  IndexMode=Zero-based  InputPortWidth=8  IndexOptions=Index vector (dialog)  Indices=6  OutputSizes=1
  Selector4 : Selector  IndexMode=Zero-based  InputPortWidth=8  IndexOptions=Index vector (dialog)  Indices=7  OutputSizes=1
  Selector5 : Selector  IndexMode=Zero-based  InputPortWidth=8  IndexOptions=Index vector (dialog)  Indices=0  OutputSizes=1
  Selector6 : Selector  IndexMode=Zero-based  InputPortWidth=8  IndexOptions=Index vector (dialog)  Indices=1  OutputSizes=1
  Selector7 : Selector  IndexMode=Zero-based  InputPortWidth=8  IndexOptions=Index vector (dialog)  Indices=2  OutputSizes=1
  Selector8 : Selector  IndexMode=Zero-based  InputPortWidth=8  IndexOptions=Index vector (dialog)  Indices=3  OutputSizes=1
  Shift Arithmetic : ArithShift  BitShiftNumber=8  BitShiftDirection=Left
  Shift Arithmetic1 : ArithShift  BitShiftNumber=16  BitShiftDirection=Left
  Shift Arithmetic2 : ArithShift  BitShiftNumber=24  BitShiftDirection=Left
  Shift Arithmetic3 : ArithShift  BitShiftNumber=8  BitShiftDirection=Left
  Shift Arithmetic4 : ArithShift  BitShiftNumber=8  BitShiftDirection=Left
  wires:
  Selector3/1 -> Data Type Conversion2/1
  Shift Arithmetic/1 -> Add/2
  Shift Arithmetic2/1 -> Add/4
  Data Type Conversion/1 -> Add/1
  Selector1/1 -> Data Type Conversion/1
  Selector4/1 -> Data Type Conversion3/1
  Add/1 -> Data Store Write2/1
  Shift Arithmetic1/1 -> Add/3
  Selector2/1 -> Data Type Conversion1/1
  Selector5/1 -> Data Type Conversion7/1
  Selector8/1 -> Data Type Conversion4/1
  Data Type Conversion4/1 -> Shift Arithmetic4/1
  Data Type Conversion6/1 -> Add1/1
  Selector7/1 -> Data Type Conversion6/1
  Selector6/1 -> Data Type Conversion5/1
  In1/1 -> Selector3/1, Selector4/1, Selector2/1, Selector1/1, Selector5/1, Selector6/1, Selector7/1, Selector8/1
  Add1/1 -> Data Type Conversion8/1
  Data Type Conversion1/1 -> Shift Arithmetic/1
  Data Type Conversion2/1 -> Shift Arithmetic1/1
  Data Type Conversion3/1 -> Shift Arithmetic2/1
  Data Type Conversion5/1 -> Shift Arithmetic3/1
  Shift Arithmetic4/1 -> Add1/2
  Shift Arithmetic3/1 -> Add2/2
  Data Type Conversion7/1 -> Add2/1
  Add2/1 -> Data Type Conversion9/1
  Data Type Conversion8/1 -> Data Store Write1/1
  Data Type Conversion9/1 -> Data Store Write3/1
